simulink model "punto_10"  (R2022a)
settings: Solver=VariableStepAuto  StartTime=0.0  StopTime=10.0  RelTol=1e-3
undefined symbols (not defined in the file): A, B
libraries: dspvision x1
settings Model: Creator=mac  LastModifiedBy=mac

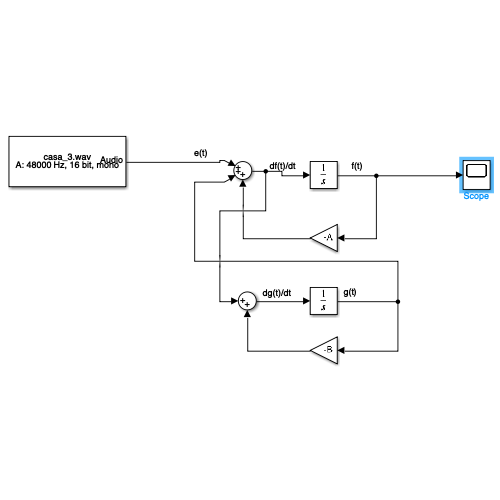
[thumbnail: Simulink's stored preview of the top-level diagram]
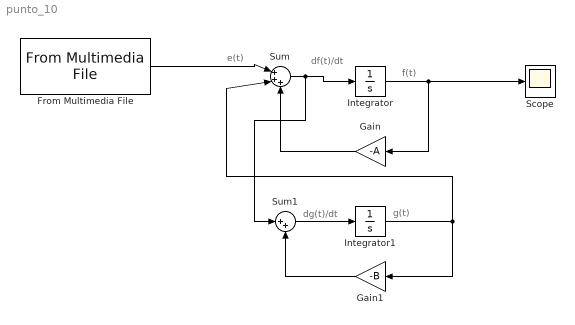
== system punto_10 ==
  note: df(t)/dt
  note: e(t)
  note: f(t)
  note: g(t)
  note: dg(t)/dt
  From Multimedia File : dspvision/From Multimedia File  inputFilename=/Users/mac/Documents/Juan Manuel/UR/2022-2/Señales/casa_3.wav  readRange=[1 Inf]  loop=on  numPlays=inf  outputStreams=Audio only  videoDataType=single  audioDataType=double  inheritSampleTime=on  userDefinedSampleTime=1/30  noAudioOutput=off  isIntensityVideo=off  fourcc=RGB  colorVideoFormat=Separate color signals  outputEOF=off  dataOrg=Column-major  audioFrameSize=1  computeAudioFrameSize=off  outSamplingMode=Sample based
  Gain : Gain  Gain=-A
  Gain1 : Gain  Gain=-B
  Integrator : Integrator
  Integrator1 : Integrator
  Scope : Scope
  Sum : Sum  Inputs=|+++
  Sum1 : Sum  Inputs=|++
  wires:
  Gain/1 -> Sum/3
  Sum/1 -> Sum1/1, Integrator/1
  Integrator1/1 -> Sum/2, Gain1/1
  Integrator/1 -> Scope/1, Gain/1
  From Multimedia File/1 -> Sum/1
  Gain1/1 -> Sum1/2
  Sum1/1 -> Integrator1/1
